simulink model "Noa_Nofusion_angle"  (R2020b)
settings: Solver=FixedStepDiscrete  StartTime=0.0  StopTime=Inf  FixedStep=0.01  RelTol=1e-3
PostLoadFcn:
  | if any(exist('dsrtsu_mdlpostloadfcn', 'file') ~= 0), dsrtsu_mdlpostloadfcn('Execute', bdroot); end
InitFcn:
  | , if any(exist('rtifpga_mdlclblib', 'file') ~= 0), rtifpga_mdlclblib('Init', bdroot); end,
  | , if any(exist('dsmpb_private', 'file') ~= 0), dsmpb_private('dsmpb_mdlclblib', 'Init', bdroot); end,
undefined symbols (not defined in the file): ACC_TimeGap_DecSetSwt, ACC_TimeGap_IncSetSwt, AccelPedalPosn, AccelPedalPosnVldty, AccelPedlPosnDiagc, AccPedalOverride, ACU_ShiftInProgress, ADAS_Posn_CurLane, AESSwtReq, ALC_SwtReq, BrkPedalSts, CC_ACC_CANCEL_OFFSwt, CC_ACC_CRUISE_OFFSwt, CC_ACC_DecSetSpd_SetSwt, CC_ACC_IncSetSpd_ResuSwt, CC_ACCSwtErr, CharSpd_ms, CSA_NODE, CURRENT_GEAR, CurrentGearValid, DiscIntNeverNeededParam, DrvDoorSts, DrvSBR, DrvTrqReqOvld, ECMACCInterface, ECMRespACC, ELKSwtReq, EngLimpHomeSts, EngSpd, EngState, EngState_PHEV, EngTrqMaxActSpd, EngTrqMinAct, EPS_DrvInpTrqVal_HighReslolution, EPS_FailSts, EPS_LKATorqOvrlDlvd, EPS_LKATorqOvrlDlvdVld, EPS_LKATrqOvlDlvdSts, EPS_SteerMod, EPS_TrqSnsrSts, EQ4_APPINFO, EQ4_LA_ELEM, EQ4_LA_HDR, EQ4_LAP_ELEM, EQ4_LAP_HDR, EQ4_LH_ELEM, EQ4_LH_HDR, EQ4_LRE_ELEM, EQ4_LRE_HDR, ESS_PedSwtReq, ESS_VehSwtReq, FFogLmpSts_F_Pbox, FLWheelDriveDirection, FLWheelSpd, FrntWiprSwtSts, FrntWshrSwtSts, FRWheelDriveDirection, FRWheelSpd, HazardLmpSwtSts, HCU_AccelPedalPosn_Diag ... (+151)
libraries: simulink x138, dsmpblib x33, canfdmsglib x10
(part 4 of 17)

== system Noa_Nofusion_angle/Common ==
  note: VIE
      | (VehicleInfomationEvaluation)
  note: CAL
      | (ConfigurationCalibration)
  note: DMS
      | (DriverMonitorSystem)
  note: EHR
      | (ElectronicHorizonReconstructor)
  IfCANBus : Inport
  function : TriggerPort  TriggerType=function-call  VariantControl=Variant
  Bus Assignment1 : BusAssignment  AssignedSignals=SteerWheelAngSign,SteerWheelAng,SteerWheelSpd,SAS_Sts
  Bus Assignment2 : BusAssignment  AssignedSignals=FLWheelSpd,FRWheelSpd,RLWheelSpd,RRWheelSpd,FLWheelDriveDirection,FRWheelDriveDirection,RLWheelDriveDirection,RRWheelDriveDirection,VehStandstill
  Bus Assignment3 : BusAssignment  AssignedSignals=VehLgtAccel,VehYawRate
  Bus Creator : BusCreator  Inputs=11
  Bus Creator2 : BusCreator  Commented=on  Inputs=6
  Bus Creator3 : BusCreator  Inputs=4
  Bus Creator4 : BusCreator  Inputs=3
  Bus Selector : BusSelector  OutputSignals=DMS_NODE.DMS_FD1_MSG.DMSSts,DMS_NODE.DMS_FD1_MSG.HeadDetn,DMS_NODE.DMS_FD1_MSG.DistrctnLvl_ACC,DMS_NODE.DMS_FD1_MSG.DistrctnLvlQlty_ACC,DMS_NODE.DMS_FD1_MSG.DrowsnsLvl_ACC
  Bus Selector2 : BusSelector  OutputSignals=ESP_NODE.ESP_FD3_MSG.FLWheelSpd,ESP_NODE.ESP_FD3_MSG.FRWheelSpd,ESP_NODE.ESP_FD3_MSG.RLWheelSpd,ESP_NODE.ESP_FD3_MSG.RRWheelSpd,ESP_NODE.ESP_FD3_MSG.FLWheelDriveDirection,ESP_NODE.ESP_FD3_MSG.FRWheelDriveDirection,ESP_NODE.ESP_FD3_MSG.RLWheelDriveDirection,ESP_NODE.ESP_FD3_MSG.RRWheelDriveDirection,ESP_NODE.ESP_FD2_MSG.VehStandstill
  Bus Selector3 : BusSelector  OutputSignals=CSA_NODE.CSA2_MSG.SteerWheelAngSign,CSA_NODE.CSA2_MSG.SteerWheelAng,CSA_NODE.CSA2_MSG.SteerWheelSpd,CSA_NODE.CSA2_MSG.SAS_Sts
  Bus Selector4 : BusSelector  OutputSignals=ABM_NODE.ABM2_MSG.VehLgtAccel,ABM_NODE.ABM2_MSG.VehYawRate
  Bus Selector8 : BusSelector  Commented=on  OutputSignals=ESP_NODE.ESP_FD2_MSG.VehSpd
  CAL : Subsystem
  Constant1 : Constant  Value=0  OutDataTypeStr=Bus: VCAN_CSA_MSG_BUS
  Constant2 : Constant  Value=0  OutDataTypeStr=Bus: VCAN_ABM_MSG_BUS
  Constant3 : Constant  Value=0  OutDataTypeStr=Bus: VCAN_ESP_MSG_BUS
  DMS : ModelReference  Commented=on  ModelNameDialog=PubIfCommonDMS_MDL.slx  SimulationMode=Normal  ModelReferenceVersion=3.0
  Data Outport : dsmpblib/Data Outport  Priority=-10000
      settings: SourceProductName=dSPACE Model Interface Blockset
  Data Outport1 : dsmpblib/Data Outport  Priority=-10000
      settings: SourceProductName=dSPACE Model Interface Blockset
  EHR : ModelReference  Commented=on  ModelNameDialog=PubIfCommonEHRV2_MDL_New.slx  SimulationMode=Normal  ModelReferenceVersion=1.4
  Ground : Ground  Commented=on
  S-Function Builder : S-Function  Commented=on  FunctionName=SWC_VIE  SFunctionModules=SWC_VIE_wrapper PubIfCommonVIE_MDL  SFunctionDeploymentMode=off  EnableBusSupport=off  mask(S-Function Builder){}
      mask help: Simulink:masks:SFunctionBuilder_MD
      mask init:
      | val = [[.9  0.75 0.75 1 1 .9 .9 1]',[1 1 0.75 0.75 .9 .9 1 .9]'];try , sys = get_param(gcb,'SfunBuilderFcnName');if isempty(sys), sys = get_param(gcb,'FunctionName'); end,catch, sys = get_param(gcb,'FunctionName'); end
      settings: CopyFcn=set_param(gcbh,'LinkStatus','none')  OpenFcn=sfunctionwizard(gcbh)
      mask Display: plot(val(:,1),val(:,2)),disp(sys),port_label('input',1,'arg_VIE_VCAN_ESP'),port_label('input',2,'arg_VIE_VCAN_CSA'),port_label('input',3,'arg_VIE_VCAN_ABM'),port_label('output',1,'arg_axvRefMs2'),port_label('output',2,'arg_vxvRefMs'),port_label('output',3,'arg_axvRoadSlopeMs2'),port_label('output',4,'arg_axRefMs2'),port_label('output',5,'arg_axRefDt'),port_label('output',6,'arg_psiDtOpt'),port_label('output',7,'arg_ayvRefMs2'),port_label('output',8,'arg_alpSideSlipAngle'),port_label('output',9,'arg_kapTraj'),port_label('output',10,'arg_alpSumSlideCurveness'),port_label('output',11,'arg_SteerAngleOffset_deg')
  Subsystem1 : Subsystem  Commented=on
  Subsystem2 : Subsystem  Commented=on
  Subsystem3 : Subsystem  Commented=on
  Subsystem4 : Subsystem  Commented=on
  Subsystem5 : Subsystem  Commented=on
  Subsystem6 : Subsystem  Commented=on
  Subsystem7 : Subsystem
  VIE : ModelReference  ModelNameDialog=PubIfCommonVIE_MDL.slx  SimulationMode=Normal  ModelReferenceVersion=3.6
  IfCALBus : Outport
  IfDMSBus : Outport  Port=2
  IfVIEBus : Outport  Port=3
  IfEHRBus : Outport  Port=4
  wires:
  VIE/8 -> Bus Creator/8  "alpSideSlipAngle"
  Bus Creator3/1 -> IfCALBus/1  "IfCALBus"
  VIE/6 -> Bus Creator/6  "psiDtOpt"
  CAL/2(CAL_AEB_CONFIG) -> Bus Creator3/2  "CAL_AEB_CONFIG"
  VIE/1 -> Bus Creator/1  "axvRefMs2"
  VIE/2 -> Bus Creator/2  "vxvRefMs"
  VIE/9 -> Bus Creator/9  "kapTraj"
  Bus Creator/1 -> IfVIEBus/1, Data Outport/1  "IfVIEBus"
  Bus Creator2/1 -> IfEHRBus/1  "IfEHRBus"
  Subsystem7/2(DMS_DrowsnsSts) -> Bus Creator4/2  "DrowsnsSts"
  Subsystem7/1(DMS_DistractnSts) -> Bus Creator4/1  "DistractnSts"
  IfCANBus/1 -> [IfCANBus]
  [IfCANBus] -> Bus Selector/1
  VIE/4 -> Bus Creator/4  "axRefMs2"
  Bus Creator4/1 -> IfDMSBus/1, Data Outport1/1  "IfDMSBus"
  VIE/7 -> Bus Creator/7  "ayvRefMs2"
  CAL/3(NvMReadWriteU8) -> Bus Creator3/3  "NvMReadWriteU8"
  CAL/4(CAL_AHBC_CONFIG) -> Bus Creator3/4  "CAL_AHBC_CONFIG"
  Subsystem7/3(DMS_DriverSts) -> Bus Creator4/3  "DriverSts"
  VIE/10 -> Bus Creator/10  "alpSumSlideCurveness"
  VIE/3 -> Bus Creator/3  "axvRoadSlopeMs2"
  VIE/5 -> Bus Creator/5  "axRefDt"
  CAL/1(CAL_VSM_CONFIG) -> Bus Creator3/1  "CAL_VSM_CONFIG"
  VIE/11 -> Bus Creator/11  "SteerAngleOffset_deg"
  Subsystem1/1(EHRV2_VCAN_POSN) -> EHR/1
  Subsystem3/1(EHRV2_VCAN_STUB) -> EHR/3
  Subsystem5/1(EHRV2_VCAN_SEG) -> EHR/2
  Subsystem4/1(EHRV2_VCAN_PROFLONG) -> EHR/5
  Subsystem2/1(EHRV2_VCAN_PROFSHORT) -> EHR/4
  Subsystem6/1(EHRV2_VCAN_META) -> EHR/6
  Bus Selector8/1 -> EHR/7  "<VehSpd>"
  Ground/1 -> EHR/8
  [IfCANBus] -> Bus Selector8/1, Subsystem6/1(In1), Subsystem4/1(In1), Subsystem2/1(In1), Subsystem3/1(In1), Subsystem5/1(In1), Subsystem1/1(In1)
  Bus Selector/1 -> Subsystem7/1(DMSSts)  "<DMSSts>"
  Bus Selector/2 -> Subsystem7/2(HeadDetn)  "<HeadDetn>"
  Bus Selector/3 -> Subsystem7/3(DistrctnLvl_ACC)  "<DistrctnLvl_ACC>"
  Bus Selector/4 -> Subsystem7/4(DistrctnLvlQlty_ACC)  "<DistrctnLvlQlty_ACC>"
  Bus Selector/5 -> Subsystem7/5(DrowsnsLvl_ACC)  "<DrowsnsLvl_ACC>"
  [IfCANBus] -> Bus Selector4/1, Bus Selector3/1, Bus Selector2/1
  EHR/1 -> Bus Creator2/1  "EHRV2_HDR"
  EHR/2 -> Bus Creator2/2  "EHRV2_HutHandshake"
  EHR/3 -> Bus Creator2/3  "EHRV2_ROAD_ROI"
  EHR/4 -> Bus Creator2/4  "EHRV2_ROAD_INFO"
  EHR/5 -> Bus Creator2/5  "EHRV2_NAV_INFO"
  EHR/6 -> Bus Creator2/6  "EHRV2_DYNAMIC_INFO"
  Constant3/1 -> Bus Assignment2/1
  Bus Selector2/1 -> Bus Assignment2/2  "<FLWheelSpd>"
  Bus Selector2/2 -> Bus Assignment2/3  "<FRWheelSpd>"
  Bus Selector2/3 -> Bus Assignment2/4  "<RLWheelSpd>"
  Bus Selector2/4 -> Bus Assignment2/5  "<RRWheelSpd>"
  Bus Selector2/5 -> Bus Assignment2/6  "<FLWheelDriveDirection>"
  Bus Selector2/6 -> Bus Assignment2/7  "<FRWheelDriveDirection>"
  Bus Selector2/7 -> Bus Assignment2/8  "<RLWheelDriveDirection>"
  Bus Selector2/8 -> Bus Assignment2/9  "<RRWheelDriveDirection>"
  Bus Selector2/9 -> Bus Assignment2/10  "<VehStandstill>"
  Bus Assignment2/1 -> VIE/1
  Constant1/1 -> Bus Assignment1/1
  Bus Selector3/1 -> Bus Assignment1/2  "<SteerWheelAngSign>"
  Bus Selector3/2 -> Bus Assignment1/3  "<SteerWheelAng>"
  Bus Selector3/3 -> Bus Assignment1/4  "<SteerWheelSpd>"
  Bus Selector3/4 -> Bus Assignment1/5  "<SAS_Sts>"
  Bus Assignment1/1 -> VIE/2
  Constant2/1 -> Bus Assignment3/1
  Bus Selector4/1 -> Bus Assignment3/2  "<VehLgtAccel>"
  Bus Selector4/2 -> Bus Assignment3/3  "<VehYawRate>"
  Bus Assignment3/1 -> VIE/3

== system Noa_Nofusion_angle/Control1 ==
  note: VMC-LAT
      | (LateralControl)
  note: VMC-LON
      | (LongtitudeControl)
  IfVCANBus : Inport  OutDataTypeStr=Bus: VCAN_BUS
  IfVSMBus : Inport  Port=2
  IfTOSBus : Inport  Port=3
  IfRFMBus : Inport  Port=4
  IfEHRBus : Inport  Port=5
  IfVIEBus : Inport  Port=6
  IfRoadBus : Inport  Port=7
  IfPlanbus : Inport  Port=8
  roadwidth : Inport  Port=9
  function : TriggerPort  TriggerType=function-call  VariantControl=Variant
  Bus Assignment : BusAssignment  AssignedSignals=dCurrentLaneWidth
  Bus Assignment1 : BusAssignment  AssignedSignals=CURRENT_GEAR,SHIFT_IN_PROGRESS
  Bus Assignment2 : BusAssignment  AssignedSignals=NoBrkForce,VehStandstill
  Bus Assignment4 : BusAssignment  AssignedSignals=ACU_ShiftInProgress,HCU_PTDrvMod,TotWheelTrq,MinPsblWheelTrq
  Bus Creator1 : BusCreator  Inputs=3
  Bus Creator2 : BusCreator  Inputs=4
  Bus Creator3 : BusCreator  Inputs=4
  Bus Selector : BusSelector  OutputSignals=PLAN_ACCPLAN,PLAN_Longctrl_DecelToStopReq
  Bus Selector1 : BusSelector  OutputSignals=vxvRefMs,axvRefMs2,ayvRefMs2,kapTraj,alpSideSlipAngle,psiDtOpt,SteerAngleOffset_deg
  Bus Selector11 : BusSelector  OutputSignals=RFM_ROAD
  Bus Selector13 : BusSelector  OutputSignals=DCT_NODE.DCT5_MSG.CURRENT_GEAR,DCT_NODE.DCT5_MSG.SHIFT_IN_PROGRESS
  Bus Selector2 : BusSelector  OutputSignals=EPS_NODE.EPS_FD1_MSG.EPS_SteerMod,EPS_NODE.EPS_FD1_MSG.EPS_DrvInpTrqVal_HighReslolution,EPS_NODE.EPS_FD1_MSG.EPS_LKATorqOvrlDlvd,EPS_NODE.EPS_FD1_MSG.EPS_LKATorqOvrlDlvdVld
  Bus Selector3 : BusSelector  OutputSignals=vxvRefMs,axvRoadSlopeMs2,axRefMs2,alpSideSlipAngle,axRefDt
  Bus Selector4 : BusSelector  OutputSignals=CSA_NODE.CSA2_MSG.SteerWheelAng,CSA_NODE.CSA2_MSG.SteerWheelAngSign,CSA_NODE.CSA2_MSG.SteerWheelSpd,CSA_NODE.CSA2_MSG.SteerWheelSpdSign
  Bus Selector5 : BusSelector  OutputSignals=ESP_NODE.ESP_FD2_MSG.NoBrkForce,ESP_NODE.ESP_FD2_MSG.VehStandstill
  Bus Selector6 : BusSelector  OutputSignals=VSM_LAT_CTRL
  Bus Selector7 : BusSelector  OutputSignals=HCU_NODE.HCU_FD1_MSG.ACU_ShiftInProgress,HCU_NODE.HCU_FD3_MSG.HCU_PTDrvMod,HCU_NODE.HCU_FD1_MSG.TotWheelTrq,HCU_NODE.HCU_FD1_MSG.MinPsblWheelTrq
  Bus Selector8 : BusSelector  OutputSignals=VSM_LON_CTRL
  Bus Creator : BusCreator  Inputs=4
  Constant1 : Constant  Value=0  OutDataTypeStr=Bus: VCAN_DCT_MSG_BUS
  Constant3 : Constant  Value=0  OutDataTypeStr=Bus: VCAN_ESP_MSG_BUS
  Constant4 : Constant  Value=0  OutDataTypeStr=Bus: VCAN_HCU_MSG_BUS
  Data Type Conversion : DataTypeConversion
  LATC : ModelReference  ModelNameDialog=PubIfControlLATC_MDL.slx  SimulationMode=Normal  ModelReferenceVersion=3.279
  LON : ModelReference  ModelNameDialog=PubIfControlLONC_MDL.slx  SimulationMode=Normal  ModelReferenceVersion=3.54
  Signal Copy : SignalConversion  OverrideOpt=off
  Subsystem : Subsystem
  Terminator : Terminator
  Terminator2 : Terminator
  IfLONBus : Outport
  IfLATBus : Outport  Port=2
  wires:
  IfVIEBus/1 -> Bus Selector3/1, Bus Selector1/1
  Bus Creator1/1 -> IfLONBus/1  "IfLONBus"
  IfVCANBus/1 -> Bus Selector7/1, Subsystem/1(In1), Bus Selector13/1, Bus Selector5/1, Bus Selector4/1, Bus Selector2/1
  IfVSMBus/1 -> Bus Selector8/1, Bus Selector6/1
  IfRoadBus/1 -> Bus Selector11/1
  Bus Selector11/1 -> Bus Assignment/1  "<RFM_ROAD>"
  Bus Selector1/7 -> LATC/8  "<SteerAngleOffset_deg>"
  Bus Selector2/3 -> Bus Creator2/3  "<EPS_LKATorqOvrlDlvd>"
  Bus Selector2/2 -> Bus Creator2/2  "<EPS_DrvInpTrqVal_HighReslolution>"
  Bus Selector2/4 -> Bus Creator2/4  "<EPS_LKATorqOvrlDlvdVld>"
  Bus Selector2/1 -> Bus Creator2/1  "<EPS_SteerMod>"
  Bus Creator2/1 -> LATC/9
  Bus Selector4/2 -> Bus Creator3/2  "<SteerWheelAngSign>"
  Bus Selector4/3 -> Bus Creator3/3  "<SteerWheelSpd>"
  Bus Selector4/1 -> Bus Creator3/1  "<SteerWheelAng>"
  Bus Selector4/4 -> Bus Creator3/4  "<SteerWheelSpdSign>"
  Bus Creator3/1 -> LATC/10
  LON/1 -> Bus Creator1/1  "LONC_CTRL_OUT"
  LON/3 -> Bus Creator1/3  "LONC_VLC_InternalAcc"
  Bus Selector6/1 -> LATC/1  "<VSM_LAT_CTRL>"
  Bus Selector1/1 -> LATC/2  "<vxvRefMs>"
  Bus Selector1/2 -> LATC/3  "<axvRefMs2>"
  Bus Selector1/3 -> LATC/4  "<ayvRefMs2>"
  Bus Selector1/4 -> LATC/5  "<kapTraj>"
  Bus Selector1/5 -> Signal Copy/1  "<alpSideSlipAngle>"
  Bus Selector1/6 -> LATC/7  "<psiDtOpt>"
  IfPlanbus/1 -> Bus Selector/1
  Bus Selector3/1 -> LON/1  "<vxvRefMs>"
  Bus Selector3/2 -> LON/2  "<axvRoadSlopeMs2>"
  Bus Selector3/3 -> LON/3  "<axRefMs2>"
  Bus Selector3/4 -> LON/4  "<alpSideSlipAngle>"
  Bus Selector3/5 -> LON/5  "<axRefDt>"
  Bus Selector8/1 -> LON/10  "<VSM_LON_CTRL>"
  Bus Selector/1 -> LON/11  "<PLAN_ACCPLAN>"
  IfRFMBus/1 -> Terminator/1
  IfTOSBus/1 -> Terminator2/1
  Bus Selector/2 -> LON/12  "<PLAN_Longctrl_DecelToStopReq>"
  Constant3/1 -> Bus Assignment2/1
  Bus Assignment2/1 -> LON/6
  Bus Selector5/1 -> Bus Assignment2/2  "<NoBrkForce>"
  Bus Selector5/2 -> Bus Assignment2/3  "<VehStandstill>"
  Constant1/1 -> Bus Assignment1/1
  Bus Selector13/1 -> Bus Assignment1/2  "<CURRENT_GEAR>"
  Bus Selector13/2 -> Bus Assignment1/3  "<SHIFT_IN_PROGRESS>"
  Bus Assignment1/1 -> LON/7
  LON/2 -> Bus Creator1/2  "LONC_Hybrid_CTRL_OUT"
  Constant4/1 -> Bus Assignment4/1
  Subsystem/1(Out1) -> LON/8
  Bus Assignment4/1 -> LON/9
  Bus Selector7/1 -> Bus Assignment4/2  "<ACU_ShiftInProgress>"
  Bus Selector7/3 -> Bus Assignment4/4  "<TotWheelTrq>"
  Bus Selector7/2 -> Bus Assignment4/3  "<HCU_PTDrvMod>"
  Bus Selector7/4 -> Bus Assignment4/5  "<MinPsblWheelTrq>"
  Data Type Conversion/1 -> Bus Assignment/2
  Bus Assignment/1 -> LATC/11
  roadwidth/1 -> [roadwidth], Data Type Conversion/1
  LATC/1 -> Bus Creator/1  "IfLATBus"
  LATC/2 -> Bus Creator/2
  LATC/3 -> Bus Creator/3
  LATC/4 -> Bus Creator/4
  Bus Creator/1 -> IfLATBus/1
  Signal Copy/1 -> LATC/6

== system Noa_Nofusion_angle/EQ4_Lane_Pack1 ==
  In1 : Inport
  Bus Assignment : BusAssignment  AssignedSignals=LA_Zero_byte,LA_Protocol_Version,LA_Sync_ID,LA_Adjacent_Count
  Bus Assignment1 : BusAssignment  AssignedSignals=EQ4_LH_HDR,EQ4_LH_ELEM,EQ4_APPINFO.APP_SyncTs
  Bus Assignment2 : BusAssignment  AssignedSignals=EQ4_LRE_HDR,EQ4_LRE_ELEM
  Bus Assignment3 : BusAssignment  AssignedSignals=EQ4_LA_HDR,EQ4_LA_ELEM
  Bus Assignment4 : BusAssignment  AssignedSignals=LRE_Zero_byte,Reserved_1,LRE_CRC,LRE_Protocol_Version,LRE_Sync_ID,LRE_Count,LRE_Header_Buffer
  Bus Assignment5 : BusAssignment  AssignedSignals=LAP_Zero_byte,LAP_Protocol_Version,LAP_Sync_ID,LAP_Is_Construction_Area,LAP_Buffer_C0,LAP_INTP_Available,LAP_INTP_Count,LAP_Exit_Merge_Available,LAP_Is_Highway_Merge_Left,LAP_Is_Highway_Merge_Right,LAP_Is_Highway_Exit_Left,LAP_Is_Highway_Exit_Right,LAP_Vertical_Surface_Available,LAP_Vertical_Surface_VR_End,Reserved_1,LAP_Vertical_Surface_C0,LAP_Vertical_Surface_C1,LAP_Vertical_Surface_C2,LAP_Vertical_Surface_C3,LAP_Path_Pred_CRC,LAP_Path_Pred_Available,LAP_Path_Pred_First_Valid,LAP_Path_Pred_Second_Valid,LAP_Path_Pred_Half_Width,LAP_Path_Pred_Conf,LAP_Is_Triggered_SDM_Model,Reserved_2,LAP_Path_Pred_First_VR_End,LAP_Path_Pred_second_VR_End,Reserved_3,LAP_Path_Pred_First_C0,LAP_Path_Pred_First_C1,LAP_Path_Pred_First_C2,LAP_Path_Pred_First_C3,LAP_Path_Pred_Second_C0,LAP_Path_Pred_Second_C1,LAP_Path_Pred_Second_C2,LAP_Path_Pred_Second_C3
  Bus Assignment6 : BusAssignment  AssignedSignals=LH_Zero_byte,LH_Protocol_Version,LH_Sync_ID,LH_Lanes_Count,Reserved_1,LH_Estimated_Width,Reserved_2
  Bus Assignment7 : BusAssignment  AssignedSignals=EQ4_LAP_HDR,EQ4_LAP_ELEM
  Bus Selector : BusSelector  OutputSignals=EQ4_LA.EQ4_LA_HDR,EQ4_LA.EQ4_LA_ELEM,EQ4_LA.EQ4_APPINFO.H
  Bus Selector1 : BusSelector  OutputSignals=EQ4_LH.EQ4_LH_HDR,EQ4_LH.EQ4_LH_ELEM,EQ4_LH.EQ4_APPINFO.H
  Bus Selector2 : BusSelector  OutputSignals=EQ4_LRE.EQ4_LRE_HDR,EQ4_LRE.EQ4_LRE_ELEM,EQ4_LRE.EQ4_APPINFO.H
  Bus Selector3 : BusSelector  OutputSignals=LA_Zero_byte,LA_Protocol_Version,LA_Sync_ID,LA_Adjacent_Count
  Bus Selector4 : BusSelector  OutputSignals=LRE_Zero_byte,Reserved_1,LRE_CRC,LRE_Protocol_Version,LRE_Sync_ID,LRE_Count,LRE_Header_Buffer
  Bus Selector5 : BusSelector  OutputSignals=LH_Zero_byte,LH_Protocol_Version,LH_Sync_ID,LH_Lanes_Count,Reserved_1,LH_Estimated_Width,Reserved_2
  Bus Selector6 : BusSelector  OutputSignals=EQ4_LAP.EQ4_LAP_HDR,EQ4_LAP.EQ4_LAP_ELEM,EQ4_LAP.EQ4_APPINFO.H
  Bus Selector7 : BusSelector  OutputSignals=LAP_Zero_byte,LAP_Protocol_Version,LAP_Sync_ID,LAP_Is_Construction_Area,LAP_Buffer_C0,LAP_INTP_Available,LAP_INTP_Count,LAP_Exit_Merge_Available,LAP_Is_Highway_Merge_Left,LAP_Is_Highway_Merge_Right,LAP_Is_Highway_Exit_Left,LAP_Is_Highway_Exit_Right,LAP_Vertical_Surface_Available,LAP_Vertical_Surface_VR_End,Reserved_1,LAP_Vertical_Surface_C0,LAP_Vertical_Surface_C1,LAP_Vertical_Surface_C2,LAP_Vertical_Surface_C3,LAP_Path_Pred_CRC,LAP_Path_Pred_Available,LAP_Path_Pred_First_Valid,LAP_Path_Pred_Second_Valid,LAP_Path_Pred_Half_Width,LAP_Path_Pred_Conf,LAP_Is_Triggered_SDM_Model,Reserved_2,LAP_Path_Pred_First_VR_End,LAP_Path_Pred_second_VR_End,Reserved_3,LAP_Path_Pred_First_C0,LAP_Path_Pred_First_C1,LAP_Path_Pred_First_C2,LAP_Path_Pred_First_C3,LAP_Path_Pred_Second_C0,LAP_Path_Pred_Second_C1,LAP_Path_Pred_Second_C2,LAP_Path_Pred_Second_C3
  Constant1 : Constant  Value=0  OutDataTypeStr=Bus: EQ4_LA_BUS
  Constant2 : Constant  Value=0  OutDataTypeStr=Bus: EQ4_LH_BUS
  Constant3 : Constant  Value=0  OutDataTypeStr=Bus: EQ4_LRE_BUS
  Constant4 : Constant  Value=0  OutDataTypeStr=Bus: EQ4_LA_HDR_BUS
  Constant5 : Constant  Value=0  OutDataTypeStr=Bus: EQ4_LRE_HDR_BUS
  Constant6 : Constant  Value=0  OutDataTypeStr=Bus: EQ4_LAP_BUS
  Constant7 : Constant  Value=0  OutDataTypeStr=Bus: EQ4_LH_HDR_BUS
  Constant8 : Constant  Value=0  OutDataTypeStr=Bus: EQ4_LAP_HDR_BUS
  Data Type Conversion{,1..4} (5 alike) : DataTypeConversion
  For Each Subsystem1 : Subsystem  TreatAsAtomicUnit=on
  For Each Subsystem2 : Subsystem  TreatAsAtomicUnit=on
  For Each Subsystem3 : Subsystem  TreatAsAtomicUnit=on
  For Each Subsystem4 : Subsystem  TreatAsAtomicUnit=on
  EQ4_LAP : Outport
  EQ4_LA : Outport  Port=2
  EQ4_LH : Outport  Port=3
  EQ4_LRE : Outport  Port=4
  wires:
  In1/1 -> Bus Selector2/1, Bus Selector1/1, Bus Selector6/1, Bus Selector/1
  Bus Assignment2/1 -> EQ4_LRE/1  "mcuEQ4_LRE"
  Constant2/1 -> Bus Assignment1/1
  Bus Assignment1/1 -> EQ4_LH/1  "mcuEQ4_LH"
  Constant3/1 -> Bus Assignment2/1
  Bus Assignment3/1 -> EQ4_LA/1  "mcuEQ4_LA"
  Bus Selector/1 -> Bus Selector3/1  "<EQ4_LA_HDR>"
  Bus Selector/2 -> For Each Subsystem3/1(In1)  "<EQ4_LA_ELEM>"
  Bus Selector1/1 -> Bus Selector5/1  "<EQ4_LH_HDR>"
  Bus Selector1/2 -> For Each Subsystem1/1(In1)  "<EQ4_LH_ELEM>"
  Bus Selector2/1 -> Bus Selector4/1  "<EQ4_LRE_HDR>"
  Bus Selector2/2 -> For Each Subsystem2/1(In1)  "<EQ4_LRE_ELEM>"
  Constant1/1 -> Bus Assignment3/1
  Constant4/1 -> Bus Assignment/1
  Bus Assignment/1 -> Bus Assignment3/2
  Bus Selector3/1 -> Bus Assignment/2  "<LA_Zero_byte>"
  Bus Selector3/2 -> Bus Assignment/3  "<LA_Protocol_Version>"
  Bus Selector3/4 -> Bus Assignment/5  "<LA_Adjacent_Count>"
  Constant5/1 -> Bus Assignment4/1
  Bus Selector4/6 -> Bus Assignment4/7  "<LRE_Count>"
  Bus Selector4/7 -> Bus Assignment4/8  "<LRE_Header_Buffer>"
  Bus Selector4/4 -> Bus Assignment4/5  "<LRE_Protocol_Version>"
  Bus Selector4/3 -> Bus Assignment4/4  "<LRE_CRC>"
  Bus Selector4/2 -> Bus Assignment4/3  "<Reserved_1>"
  Bus Selector4/1 -> Bus Assignment4/2  "<LRE_Zero_byte>"
  Bus Assignment4/1 -> Bus Assignment2/2
  Constant7/1 -> Bus Assignment6/1
  Bus Assignment6/1 -> Bus Assignment1/2
  Bus Selector5/6 -> Bus Assignment6/7  "<LH_Estimated_Width>"
  Bus Selector5/5 -> Bus Assignment6/6  "<Reserved_1>"
  Bus Selector5/7 -> Bus Assignment6/8  "<Reserved_2>"
  Bus Selector5/4 -> Bus Assignment6/5  "<LH_Lanes_Count>"
  Bus Selector5/2 -> Bus Assignment6/3  "<LH_Protocol_Version>"
  Bus Selector5/1 -> Bus Assignment6/2  "<LH_Zero_byte>"
  For Each Subsystem1/1(Out1) -> Bus Assignment1/3
  For Each Subsystem2/1(Out1) -> Bus Assignment2/3
  For Each Subsystem3/1(Out1) -> Bus Assignment3/3
  Bus Selector1/3 -> Data Type Conversion2/1, Data Type Conversion/1  "<H>"
  Data Type Conversion/1 -> Bus Assignment1/4
  Bus Selector/3 -> Data Type Conversion1/1  "<H>"
  Data Type Conversion1/1 -> Bus Assignment/4
  Data Type Conversion2/1 -> Bus Assignment6/4
  Data Type Conversion3/1 -> Bus Assignment4/6
  Bus Selector2/3 -> Data Type Conversion3/1  "<H>"
  Data Type Conversion4/1 -> Bus Assignment5/4
  For Each Subsystem4/1(Out1) -> Bus Assignment7/3
  Bus Assignment5/1 -> Bus Assignment7/2
  Constant8/1 -> Bus Assignment5/1
  Constant6/1 -> Bus Assignment7/1
  Bus Selector6/2 -> For Each Subsystem4/1(In1)  "<EQ4_LAP_ELEM>"
  Bus Assignment7/1 -> EQ4_LAP/1  "mcuEQ4_LAP"
  Bus Selector6/3 -> Data Type Conversion4/1  "<H>"
  Bus Selector6/1 -> Bus Selector7/1  "<EQ4_LAP_HDR>"
  Bus Selector7/1 -> Bus Assignment5/2  "<LAP_Zero_byte>"
  Bus Selector7/2 -> Bus Assignment5/3  "<LAP_Protocol_Version>"
  Bus Selector7/4 -> Bus Assignment5/5  "<LAP_Is_Construction_Area>"
  Bus Selector7/5 -> Bus Assignment5/6  "<LAP_Buffer_C0>"
  Bus Selector7/6 -> Bus Assignment5/7  "<LAP_INTP_Available>"
  Bus Selector7/7 -> Bus Assignment5/8  "<LAP_INTP_Count>"
  Bus Selector7/8 -> Bus Assignment5/9  "<LAP_Exit_Merge_Available>"
  Bus Selector7/9 -> Bus Assignment5/10  "<LAP_Is_Highway_Merge_Left>"
  Bus Selector7/10 -> Bus Assignment5/11  "<LAP_Is_Highway_Merge_Right>"
  Bus Selector7/11 -> Bus Assignment5/12  "<LAP_Is_Highway_Exit_Left>"
  Bus Selector7/12 -> Bus Assignment5/13  "<LAP_Is_Highway_Exit_Right>"
  Bus Selector7/13 -> Bus Assignment5/14  "<LAP_Vertical_Surface_Available>"
  Bus Selector7/14 -> Bus Assignment5/15  "<LAP_Vertical_Surface_VR_End>"
  Bus Selector7/15 -> Bus Assignment5/16  "<Reserved_1>"
  Bus Selector7/16 -> Bus Assignment5/17  "<LAP_Vertical_Surface_C0>"
  Bus Selector7/17 -> Bus Assignment5/18  "<LAP_Vertical_Surface_C1>"
  Bus Selector7/18 -> Bus Assignment5/19  "<LAP_Vertical_Surface_C2>"
  Bus Selector7/19 -> Bus Assignment5/20  "<LAP_Vertical_Surface_C3>"
  Bus Selector7/20 -> Bus Assignment5/21  "<LAP_Path_Pred_CRC>"
  Bus Selector7/21 -> Bus Assignment5/22  "<LAP_Path_Pred_Available>"
  Bus Selector7/22 -> Bus Assignment5/23  "<LAP_Path_Pred_First_Valid>"
  Bus Selector7/23 -> Bus Assignment5/24  "<LAP_Path_Pred_Second_Valid>"
  Bus Selector7/24 -> Bus Assignment5/25  "<LAP_Path_Pred_Half_Width>"
  Bus Selector7/25 -> Bus Assignment5/26  "<LAP_Path_Pred_Conf>"
  Bus Selector7/26 -> Bus Assignment5/27  "<LAP_Is_Triggered_SDM_Model>"
  Bus Selector7/27 -> Bus Assignment5/28  "<Reserved_2>"
  Bus Selector7/28 -> Bus Assignment5/29  "<LAP_Path_Pred_First_VR_End>"
  Bus Selector7/29 -> Bus Assignment5/30  "<LAP_Path_Pred_second_VR_End>"
  Bus Selector7/30 -> Bus Assignment5/31  "<Reserved_3>"
  Bus Selector7/31 -> Bus Assignment5/32  "<LAP_Path_Pred_First_C0>"
  Bus Selector7/32 -> Bus Assignment5/33  "<LAP_Path_Pred_First_C1>"
  Bus Selector7/33 -> Bus Assignment5/34  "<LAP_Path_Pred_First_C2>"
  Bus Selector7/34 -> Bus Assignment5/35  "<LAP_Path_Pred_First_C3>"
  Bus Selector7/35 -> Bus Assignment5/36  "<LAP_Path_Pred_Second_C0>"
  Bus Selector7/36 -> Bus Assignment5/37  "<LAP_Path_Pred_Second_C1>"
  Bus Selector7/37 -> Bus Assignment5/38  "<LAP_Path_Pred_Second_C2>"
  Bus Selector7/38 -> Bus Assignment5/39  "<LAP_Path_Pred_Second_C3>"

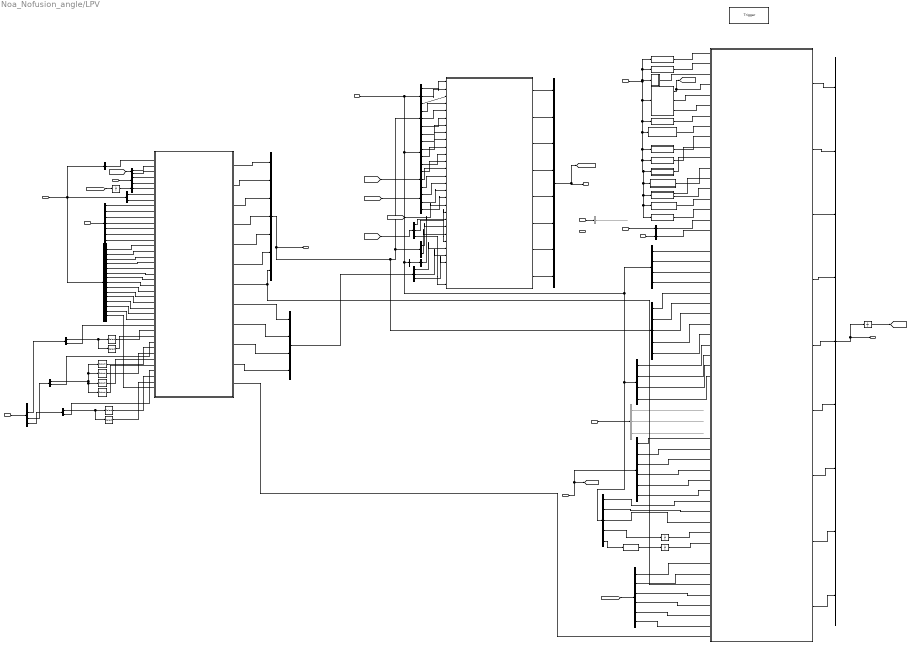
== system Noa_Nofusion_angle/LPV ==
  FaultRnk : Inport
  FaultTriggers : Inport  Port=2
  IfALLBus : Inport  Port=3
  IfCANBus : Inport  Port=4
  IfCALBus : Inport  Port=5
  IfDMSBus : Inport  Port=6
  IfEHRBus : Inport  Port=7
  IfVIEBus : Inport  Port=8
  IfEQ4Bus : Inport  Port=9
  RFM_LANES : Inport  Port=10
  function : TriggerPort  TriggerType=function-call  VariantControl=Variant
  ABM_Pack : Subsystem
  BCM_Pack : Subsystem
  Bus Creator : BusCreator  Inputs=9
  Bus Creator1 : BusCreator  Inputs=8
  Bus Creator3 : BusCreator  Inputs=4
  Bus Creator9 : BusCreator  Inputs=7
  Bus Selector : BusSelector  OutputSignals=LSM_UpdateCnt,LSM_TJA_ICA,LSM_HWA,LSM_LCK,LSM_ESS
  Bus Selector1 : BusSelector  OutputSignals=signal1.TOS_P0_TARGET_LINE
  Bus Selector10 : BusSelector  OutputSignals=LSM_HWA,LSM_ESS,LSM_UpdateCnt
  Bus Selector12 : BusSelector  OutputSignals=VSM_LON_CTRL
  Bus Selector13 : BusSelector  OutputSignals=LSM_PilotSPLDist,LSM_PilotSPL,LSM_PilotRoadSts
  Bus Selector14 : BusSelector  OutputSignals=PLAN_ALC_DECS
  Bus Selector15 : BusSelector  OutputSignals=EQ4_LA_ELEM,EQ4_LA_HDR
  Bus Selector16 : BusSelector  OutputSignals=PLAN_ACCPLAN,PLAN_DriverOffConditionFulfilled,PLAN_ALC_DECS,PLAN_DPC_ESS,PLAN_NOH_SetSpdAdjReq,PLAN_NOH_SetSpdAdjVal
  Bus Selector17 : BusSelector  OutputSignals=EQ4_LH_ELEM,EQ4_LH_HDR
  Bus Selector18 : BusSelector  OutputSignals=VSM_HMI,VSM_UOM_LC_BUS,MRCReq
  Bus Selector19 : BusSelector  OutputSignals=DriverSts
  Bus Selector2 : BusSelector  OutputSignals=vxvRefMs,kapTraj
  Bus Selector20 : BusSelector  OutputSignals=CAL_VSM_CONFIG
  Bus Selector21 : BusSelector  OutputSignals=lanebus.RFM_LINE_L1,lanebus.RFM_LINE_R1,lanebus.RFM_LINE_LB,lanebus.RFM_LINE_RB
  Bus Selector22 : BusSelector  Commented=on  OutputSignals=EHRV2_HDR,EHRV2_ROAD_ROI,EHRV2_ROAD_INFO
  Bus Selector23 : BusSelector  OutputSignals=axvRefMs2,vxvRefMs,axvRoadSlopeMs2,axRefDt,ayvRefMs2,kapTraj
  Bus Selector24 : BusSelector  OutputSignals=aebbus.AEB_IPHUT_INFO,aebbus.AEB_BRK_INFO,roadbus.RFM_TSR,latbus.LATC_IFCAngCmdReqValue,latbus.LATC_IFCFuncAngCmdReqFlag
  Bus Selector25 : BusSelector  OutputSignals=signal1.TOS_ACCP0,signal1.TOS_AEB_LONOBJ,signal1.TOS_ELK,signal1.TOS_LCKIE
  Bus Selector26 : BusSelector  OutputSignals=EQ4_LRE_ELEM,EQ4_LRE_HDR
  Bus Selector27 : BusSelector  OutputSignals=lanebus.RFM_LINE_L1,lanebus.RFM_LINE_R1,roadbus.RFM_TSR
  Bus Selector28 : BusSelector  OutputSignals=LONC_VLC_InternalAcc
  Bus Selector29 : BusSelector  OutputSignals=LSM_PilotSts,LSM_PilotTurnSwSts
  Bus Selector3 : BusSelector  OutputSignals=lanebus.RFM_LINE_L1,lanebus.RFM_LINE_R1,lanebus.RFM_LINE_L2,lanebus.RFM_LINE_R2,lanebus.RFM_LINE_L3,lanebus.RFM_LINE_R3,lanebus.RFM_LINE_CL,lanebus.RFM_LINE_LB,lanebus.RFM_LINE_RB,lanebus.RFM_LINE_PRED,lanebus.RFM_LINEF_LB,lanebus.RFM_LINEF_RB,lanebus.RFM_LINE_ENTRY_CL,lanebus.RFM_LINE_EXIT_CL,roadbus.RFM_TSR
  Bus Selector30 : BusSelector  OutputSignals=lonbus
  Bus Selector31 : BusSelector  OutputSignals=RFM_BRANCH_LANE,RFM_LEFT_LANE,RFM_CURRENT_LANE,RFM_RIGHT_LANE,RFM_INTERSEC_ALERT,RFM_BRANCH,RFM_REC_LANES
  Bus Selector4 : BusSelector  OutputSignals=VSM_HMI,MRCReq
  Bus Selector5 : BusSelector  OutputSignals=roadbus.RFM_ROAD,roadbus.RFM_UpdateCnt
  Bus Selector6 : BusSelector  OutputSignals=signal1.TOS_LC,signal1.TOS_ACCP0,signal1.TOS_ACCP1,signal1.TOS_ACCP2,signal1.TOS_ACCP3,signal1.TOS_UpdateCnt
  Bus Selector7 : BusSelector  OutputSignals=vxvRefMs,axvRefMs2,axvRoadSlopeMs2,kapTraj
  Bus Selector8 : BusSelector  OutputSignals=EQ4_LAP,EQ4_LH,EQ4_LA,EQ4_LRE
  Bus Selector9 : BusSelector  Commented=on  OutputSignals=DFIM_VSM_STS
  CSA_Pack : Subsystem
  DCT_Pack : Subsystem
  Data Type Conversion : DataTypeConversion  OutDataTypeStr=uint8
  ECM_Pack : Subsystem
  ESP_Pack : Subsystem
  HAP_Pack : Subsystem
  HUT_Pack : Subsystem
  IfALLBus1 : InportShadow  Port=3
  IfVIEBus1 : InportShadow  Port=8
  PLAN : ModelReference  ModelNameDialog=PubIfDecisionPLAN_MDL.slx  SimulationMode=Normal  ModelReferenceVersion=1.158
  Selector : Selector  InputPortWidth=4  IndexOptions=Index vector (dialog)  Indices=1  OutputSizes=1
  Selector1 : Selector  InputPortWidth=4  IndexOptions=Index vector (dialog)  Indices=2  OutputSizes=1
  Selector2 : Selector  InputPortWidth=4  IndexOptions=Index vector (dialog)  Indices=3  OutputSizes=1
  Selector3 : Selector  InputPortWidth=4  IndexOptions=Index vector (dialog)  Indices=4  OutputSizes=1
  Selector4 : Selector  InputPortWidth=2  IndexOptions=Index vector (dialog)  Indices=1  OutputSizes=1
  Selector5 : Selector  InputPortWidth=2  IndexOptions=Index vector (dialog)  Indices=2  OutputSizes=1
  Selector6 : Selector  InputPortWidth=2  IndexOptions=Index vector (dialog)  Indices=1  OutputSizes=1
  Selector7 : Selector  InputPortWidth=2  IndexOptions=Index vector (dialog)  Indices=2  OutputSizes=1
  Subsystem : Subsystem
  Subsystem1 : Subsystem
  Subsystem2 : Subsystem
  Subsystem3 : Subsystem
  Subsystem4 : Subsystem
  Subsystem5 : Subsystem
  Unit Delay{1..4} (4 alike) : UnitDelay  SampleTime=-1  HasFrameUpgradeWarning=on
  VSM : Subsystem
  IfVSMBus : Outport
  IfLSMBus : Outport  Port=2
  IfPlanbus : Outport  Port=3
  wires:
  Bus Creator/1 -> Unit Delay4/1, IfVSMBus/1
  FaultTriggers/1 -> Bus Selector9/1
  IfCANBus/1 -> ECM_Pack/1(In1), DCT_Pack/1(In1), Subsystem4/1(In1), Subsystem3/1(In1), CSA_Pack/1(In1), HAP_Pack/1(In1), Subsystem2/1(In1), HUT_Pack/1(In1), Subsystem1/1(In1), ABM_Pack/1(In1), Subsystem/1(In1), BCM_Pack/1(In1), ESP_Pack/1(In1)
  IfDMSBus/1 -> Bus Selector19/1
  IfCALBus/1 -> Bus Selector20/1
  Bus Selector20/1 -> VSM/18(CAL_VSM_CONFIG)  "<CAL_VSM_CONFIG>"
  Bus Selector9/1 -> ?  "<DFIM_VSM_STS>"
  IfVIEBus/1 -> [IfVIEBus], Bus Selector23/1
  Bus Selector24/4 -> Unit Delay1/1  "<LATC_IFCAngCmdReqValue>"
  Bus Selector24/5 -> Data Type Conversion/1  "<LATC_IFCFuncAngCmdReqFlag>"
  Subsystem5/1(LSM_TJA_ICA) -> Bus Creator9/1  "LSM_TJA_ICA"
  Bus Selector1/1 -> Subsystem5/1(TOS_P0_TARGET_LINE)  "<TOS_P0_TARGET_LINE>"
  Subsystem5/2(LSM_LCK) -> Bus Creator9/2  "LSM_LCK"
  Bus Selector4/1 -> Subsystem5/2(VSM_HMI)  "<VSM_HMI>"
  IfEQ4Bus/1 -> Bus Selector8/1
  Subsystem5/3(LSM_HWA) -> Bus Creator9/3  "LSM_HWA"
  IfALLBus1/1 -> Bus Selector3/1, Bus Selector5/1, Bus Selector1/1
  Bus Creator9/1 -> Bus Selector10/1, Bus Selector29/1, Bus Selector/1, IfLSMBus/1  "IfLSMBus"
  Subsystem5/4(LSM_ESS) -> Bus Creator9/4  "LSM_ESS"
  Subsystem5/5(LSM_UpdateCnt) -> Bus Creator9/5  "LSM_UpdateCnt"
  [IfVSMBus] -> Bus Selector4/1
  IfVIEBus1/1 -> Bus Selector2/1
  ESP_Pack/1(VSM_VCAN_ESP) -> [ESP_Pack], VSM/4(VSM_VCAN_ESP)
  Bus Selector19/1 -> VSM/17(DriverSts)  "<DriverSts>"
  Bus Selector21/1 -> VSM/20(RFM_LINE_L1)  "<RFM_LINE_L1>"
  Bus Selector21/2 -> VSM/21(RFM_LINE_R1)  "<RFM_LINE_R1>"
  Bus Selector21/3 -> VSM/22(RFM_LINE_LB)  "<RFM_LINE_LB>"
  Bus Selector21/4 -> VSM/23(RFM_LINE_RB)  "<RFM_LINE_RB>"
  Bus Selector/1 -> VSM/24(LSM_UpdateCnt)  "<LSM_UpdateCnt>"
  Bus Selector/2 -> VSM/25(LSM_TJA_ICA)  "<LSM_TJA_ICA>"
  Bus Selector/3 -> VSM/26(LSM_HWA)  "<LSM_HWA>"
  Bus Selector/4 -> VSM/27(LSM_LCK)  "<LSM_LCK>"
  Bus Selector/5 -> VSM/28(LSM_ESS)  "<LSM_ESS>"
  Bus Selector25/1 -> VSM/29(TOS_ACCP0)  "<TOS_ACCP0>"
  Bus Selector25/2 -> VSM/30(TOS_AEB_LONOBJ)  "<TOS_AEB_LONOBJ>"
  Bus Selector25/3 -> VSM/31(TOS_ELK)  "<TOS_ELK>"
  Bus Selector25/4 -> VSM/32(TOS_LCKIE)  "<TOS_LCKIE>"
  Bus Selector22/1 -> ?  "<EHRV2_HDR>"
  Bus Selector22/2 -> ?  "<EHRV2_ROAD_ROI>"
  Bus Selector22/3 -> ?  "<EHRV2_ROAD_INFO>"
  Bus Selector23/1 -> VSM/38(axvRefMs2)  "<axvRefMs2>"
  Bus Selector23/2 -> VSM/39(vxvRefMs)  "<vxvRefMs>"
  Bus Selector23/3 -> VSM/40(axvRoadSlopeMs2)  "<axvRoadSlopeMs2>"
  Bus Selector23/4 -> VSM/41(psiDtOpt)  "<axRefDt>"
  Bus Selector23/5 -> VSM/42(ayvRefMs2)  "<ayvRefMs2>"
  Bus Selector23/6 -> VSM/43(kapTraj)  "<kapTraj>"
  Bus Selector24/1 -> VSM/44(AEB_IPHUT_INFO)  "<AEB_IPHUT_INFO>"
  Bus Selector24/2 -> VSM/45(AEB_BRK_INFO)  "<AEB_BRK_INFO>"
  Bus Selector24/3 -> VSM/46(RFM_TSR)  "<RFM_TSR>"
  Unit Delay1/1 -> VSM/47(LATC_IFCTrqOvlCmdReqValue)
  Unit Delay2/1 -> VSM/48(LATC_IFCFuncTrqCmdReqFlag)
  VSM/1(VSM_LON_CTRL) -> Bus Creator/1  "VSM_LON_CTRL"
  VSM/2(VSM_LAT_CTRL) -> Bus Creator/2  "VSM_LAT_CTRL"
  VSM/3(VSM_HMI) -> Bus Creator/3  "VSM_HMI"
  VSM/4(VSM_CTRL_LINE) -> Bus Creator/4  "VSM_CTRL_LINE"
  VSM/5(VSM_TSR) -> Bus Creator/5  "VSM_TSR"
  VSM/6(VSM_TSR_REMAIN) -> Bus Creator/6  "VSM_TSR_REMAIN"
  VSM/8(DataCLCT) -> Bus Creator/8  "DangerPlausMatrix"
  HAP_Pack/1(VSM_VCAN_HAP) -> VSM/16(VSM_VCAN_HAP)
  HUT_Pack/1(VSM_VCAN_HUT) -> VSM/13(VSM_VCAN_HUT)
  ABM_Pack/1(VSM_VCAN_ABM) -> VSM/11(VSM_VCAN_ABM)
  CSA_Pack/1(VSM_VCAN_CSA) -> VSM/10(VSM_VCAN_CSA)
  ECM_Pack/1(VSM_VCAN_ECM) -> VSM/1(VSM_VCAN_ECM)
  DCT_Pack/1(VSM_VCAN_DCT) -> VSM/2(VSM_VCAN_DCT)
  BCM_Pack/1(VSM_VCAN_BCM) -> VSM/7(VSM_VCAN_BCM)
  Subsystem3/1(VSM_VCAN_PBOX) -> VSM/9(VSM_VCAN_PBOX)
  [IfVIEBus] -> Bus Selector7/1
  [IfVSMBus] -> Bus Selector12/1
  IfEHRBus/1 -> Bus Selector22/1
  PLAN/1 -> Bus Creator1/1  "PLAN_DPC_ESS"
  PLAN/2 -> Bus Creator1/2  "PLAN_ALC_DECS"
  PLAN/3 -> Bus Creator1/3
  Bus Creator1/1 -> IfPlanbus/1, [IfPlanbus]
  [IfPlanbus] -> Unit Delay3/1
  Unit Delay3/1 -> Bus Selector14/1
  Bus Selector14/1 -> Subsystem5/6(PLAN_ALC_DECS)  "<PLAN_ALC_DECS>"
  Unit Delay4/1 -> [IfVSMBus]
  [IfPlanbus] -> Bus Selector16/1
  [IfVSMBus] -> Bus Selector18/1
  Bus Selector27/1 -> PLAN/1  "<RFM_LINE_L1>"
  Bus Selector27/2 -> PLAN/2  "<RFM_LINE_R1>"
  Bus Selector10/1 -> PLAN/4  "<LSM_HWA>"
  Bus Selector10/2 -> PLAN/5  "<LSM_ESS>"
  Bus Selector10/3 -> PLAN/6  "<LSM_UpdateCnt>"
  Bus Selector6/1 -> PLAN/7  "<TOS_LC>"
  Bus Selector6/2 -> PLAN/8  "<TOS_ACCP0>"
  Bus Selector6/3 -> PLAN/9  "<TOS_ACCP1>"
  Bus Selector6/4 -> PLAN/10  "<TOS_ACCP2>"
  Bus Selector6/5 -> PLAN/11  "<TOS_ACCP3>"
  Bus Selector6/6 -> PLAN/12  "<TOS_UpdateCnt>"
  Bus Selector27/3 -> PLAN/3  "<RFM_TSR>"
  Bus Selector12/1 -> PLAN/13  "<VSM_LON_CTRL>"
  Bus Selector30/1 -> Bus Selector28/1  "<lonbus>"
  Bus Selector7/1 -> PLAN/14  "<vxvRefMs>"
  Bus Selector7/2 -> PLAN/15  "<axvRefMs2>"
  Bus Selector7/3 -> PLAN/16  "<axvRoadSlopeMs2>"
  Bus Selector7/4 -> PLAN/17  "<kapTraj>"
  Subsystem5/6(LSM_PilotTurnSwSts) -> Bus Creator9/6  "LSM_PilotTurnSwSts"
  IfALLBus/1 -> Bus Selector30/1, Bus Selector21/1, Bus Selector24/1, Bus Selector25/1, Bus Selector6/1, Bus Selector27/1
  Subsystem5/7(LSM_PilotSts) -> Bus Creator9/7, VSM/52(LSM_PilotSts)  "LSM_PilotSts"
  VSM/7(VSM_UOM_LC) -> Bus Creator/7  "VSM_UOM_LC_BUS"
  Bus Selector18/1 -> PLAN/19  "<VSM_HMI>"
  Bus Selector18/2 -> PLAN/23  "<VSM_UOM_LC_BUS>"
  RFM_LANES/1 -> Bus Selector31/1
  Bus Selector8/3 -> Bus Selector15/1  "<EQ4_LA>"
  Bus Selector8/4 -> Bus Selector26/1  "<EQ4_LRE>"
  Bus Selector2/1 -> Subsystem5/4(vxvRefMs)  "<vxvRefMs>"
  Bus Selector2/2 -> Subsystem5/5(kapTraj)  "<kapTraj>"
  Bus Selector5/2 -> Subsystem5/8(RFM_UpdateCnt)  "<RFM_UpdateCnt>"
  Bus Selector5/1 -> Subsystem5/7(RFM_ROAD)  "<RFM_ROAD>"
  Bus Selector31/2 -> Subsystem5/10(RFM_LEFT_LANE)  "<RFM_LEFT_LANE>"
  Bus Selector31/3 -> Subsystem5/11(RFM_CURRENT_LANE)  "<RFM_CURRENT_LANE>"
  Bus Selector31/1 -> Subsystem5/9(RFM_BRANCH_LANE)  "<RFM_BRANCH_LANE>"
  Bus Selector31/4 -> Subsystem5/12(RFM_RIGHT_LANE)  "<RFM_RIGHT_LANE>"
  Bus Selector31/5 -> Subsystem5/13(RFM_INTERSEC_ALERT)  "<RFM_INTERSEC_ALERT>"
  Bus Selector31/6 -> Subsystem5/14(RFM_BRANCH)  "<RFM_BRANCH>"
  Bus Selector31/7 -> Subsystem5/15(RFM_REC_LANES)  "<RFM_REC_LANES>"
  Bus Selector3/1 -> Subsystem5/16(RFM_LINE_L1)  "<RFM_LINE_L1>"
  Bus Selector3/2 -> Subsystem5/17(RFM_LINE_R1)  "<RFM_LINE_R1>"
  Bus Selector3/3 -> Subsystem5/18(RFM_LINE_L2)  "<RFM_LINE_L2>"
  Bus Selector3/4 -> Subsystem5/19(RFM_LINE_R2)  "<RFM_LINE_R2>"
  Bus Selector3/5 -> Subsystem5/20(RFM_LINE_L3)  "<RFM_LINE_L3>"
  Bus Selector3/6 -> Subsystem5/21(RFM_LINE_R3)  "<RFM_LINE_R3>"
  Bus Selector3/7 -> Subsystem5/22(RFM_LINE_CL)  "<RFM_LINE_CL>"
  Bus Selector3/8 -> Subsystem5/23(RFM_LINE_LB)  "<RFM_LINE_LB>"
  Bus Selector3/9 -> Subsystem5/24(RFM_LINE_RB)  "<RFM_LINE_RB>"
  Bus Selector3/10 -> Subsystem5/25(RFM_LINE_PRED)  "<RFM_LINE_PRED>"
  Bus Selector3/11 -> Subsystem5/26(RFM_LINEF_LB)  "<RFM_LINEF_LB>"
  Bus Selector3/12 -> Subsystem5/27(RFM_LINEF_RB)  "<RFM_LINEF_RB>"
  Bus Selector3/13 -> Subsystem5/28(RFM_LINE_ENTRY_CL)  "<RFM_LINE_ENTRY_CL>"
  Bus Selector3/14 -> Subsystem5/29(RFM_LINE_EXIT_CL)  "<RFM_LINE_EXIT_CL>"
  Bus Selector29/1 -> PLAN/21  "<LSM_PilotSts>"
  Bus Selector29/2 -> PLAN/22  "<LSM_PilotTurnSwSts>"
  Bus Selector28/1 -> PLAN/20  "<LONC_VLC_InternalAcc>"
  [ESP_Pack] -> PLAN/18
  PLAN/4 -> Bus Creator1/4  "PLAN_HMI"
  PLAN/5 -> Bus Creator1/5
  PLAN/6 -> Bus Creator1/6
  Bus Selector16/4 -> VSM/54(PLAN_DPC_ESS)  "<PLAN_DPC_ESS>"
  Bus Selector16/3 -> VSM/53(PLAN_ALC_Decision)  "<PLAN_ALC_DECS>"
  Bus Selector16/2 -> VSM/51(PLAN_DriverOffConditionFulfilled)  "<PLAN_DriverOffConditionFulfilled>"
  Bus Selector16/1 -> VSM/50(PLAN_ACCPLAN)  "<PLAN_ACCPLAN>"
  Subsystem5/8(LSM_PilotNohExitDist) -> Bus Creator3/1
  Subsystem5/9(LSM_PilotSPLDist) -> Bus Creator3/2
  Subsystem5/10(LSM_PilotSPL) -> Bus Creator3/3
  Subsystem5/11(LSM_PilotRoadSts) -> Bus Creator3/4  "LSM_PilotRoadSts"
  Bus Creator3/1 -> Bus Selector13/1
  Bus Selector13/1 -> PLAN/24  "<LSM_PilotSPLDist>"
  Bus Selector13/2 -> PLAN/25  "<LSM_PilotSPL>"
  PLAN/7 -> Bus Creator1/7  "PLAN_NOH_SetSpdAdjReq"
  PLAN/8 -> Bus Creator1/8  "PLAN_NOH_SetSpdAdjVal"
  Bus Selector16/5 -> VSM/55(PLAN_NOH_SetSpdAdjReq)  "<PLAN_NOH_SetSpdAdjReq>"
  Bus Selector16/6 -> VSM/56(PLAN_NOH_SetSpdAdjVal)  "<PLAN_NOH_SetSpdAdjVal>"
  Bus Selector13/3 -> PLAN/26  "<LSM_PilotRoadSts>"
  ESP_Pack/2(VSM_VCAN_EPS) -> VSM/5(VSM_VCAN_EPS)
  ESP_Pack/3(VSM_VCAN_PEPS) -> VSM/6(VSM_VCAN_PEPS)
  Subsystem/1(<ACAmbTemp>) -> VSM/8(VSM_ACAmbTemp)
  Subsystem1/1(<IP_VehSpdUnit>) -> VSM/12(VSM_VCAN_IP)
  HUT_Pack/2(VSM_VCAN_CR) -> VSM/14(VSM_VCAN_CR)
  Subsystem2/1(<HighBeamSts_HC>) -> VSM/15(VSM_VCAN_HC)
  Subsystem4/1(Out1) -> VSM/3(VSM_VCAN_HCU)
  Bus Selector15/1 -> Selector/1, Selector1/1, Selector3/1, Selector2/1  "<EQ4_LA_ELEM>"
  Bus Selector15/2 -> Subsystem5/33(EQ4_LA_HDR)  "<EQ4_LA_HDR>"
  Bus Selector8/2 -> Bus Selector17/1  "<EQ4_LH>"
  Bus Selector17/1 -> Selector5/1, Selector4/1  "<EQ4_LH_ELEM>"
  Bus Selector17/2 -> Subsystem5/30(EQ4_LH_HDR)  "<EQ4_LH_HDR>"
  Selector4/1 -> Subsystem5/31(EQ4_LH_ELEM)
  Selector5/1 -> Subsystem5/32(EQ4_LH_ELEM1)
  Selector/1 -> Subsystem5/34(EQ4_LA_ELEM)
  Selector1/1 -> Subsystem5/35(EQ4_LA_ELEM1)
  Selector2/1 -> Subsystem5/36(EQ4_LA_ELEM2)
  Selector3/1 -> Subsystem5/37(EQ4_LA_ELEM3)
  Bus Selector26/2 -> Subsystem5/38(EQ4_LRE_HDR)  "<EQ4_LRE_HDR>"
  Bus Selector26/1 -> Selector7/1, Selector6/1  "<EQ4_LRE_ELEM>"
  Selector6/1 -> Subsystem5/39(EQ4_LRE_ELEM)
  Selector7/1 -> Subsystem5/40(EQ4_LRE_ELEM1)
  Bus Selector3/15 -> Subsystem5/41(RFM_TSR)  "<RFM_TSR>"
  Data Type Conversion/1 -> Unit Delay2/1
  VSM/9(VSM_MRCReq) -> Bus Creator/9
  Bus Selector18/3 -> PLAN/29  "<MRCReq>"
  Bus Selector4/2 -> Subsystem5/3(VSM_ReqMRC)  "<MRCReq>"
  Subsystem5/12(LSM_TJALineSource) -> VSM/57(LSM_TJALineSource)

== system Noa_Nofusion_angle/SensorDia ==
  function : TriggerPort  TriggerType=function-call  VariantControl=Variant
  AND : Logic  Inputs=8  IconShape=distinctive  AllPortsSameDT=off  OutDataTypeStr=boolean
  Bus Selector : BusSelector  OutputSignals=RSDS_L_hdr_TimerStempStatus Value,RSDS_R_hdr_TimerStempStatus Value,CR_L_hdr_TimerStempStatus Value,CR_R_hdr_TimerStempStatus Value,RSDS_L_hdr_ErrorStatus Value,RSDS_R_hdr_ErrorStatus Value,CR_L_hdr_ErrorStatus Value,CR_R_hdr_ErrorStatus Value
  CR_Dia : dsmpblib/Data Inport  Priority=10000
      settings: SourceProductName=dSPACE Model Interface Blockset
  Compare To Constant{,1..3} (4 alike) : simulink/Logic and Bit Operations/Compare To Constant  relop===  const=8  OutDataTypeStr=boolean
  Compare To Constant{4..7} (4 alike) : simulink/Logic and Bit Operations/Compare To Constant  relop===  const=0  OutDataTypeStr=boolean
  Signal Copy{,1..7} (8 alike) : SignalConversion  OverrideOpt=off
  Source_Dia_CRsts : Outport
  wires:
  Signal Copy6/1 -> Compare To Constant6/1  "Source_Dia_ErrorStatusCRL"
  Compare To Constant2/1 -> AND/3
  Compare To Constant7/1 -> AND/8
  Bus Selector/7 -> Signal Copy6/1  "<CR_L_hdr_ErrorStatus Value>"
  Compare To Constant6/1 -> AND/7
  AND/1 -> Source_Dia_CRsts/1  "Source_Dia_CRsts"
  Compare To Constant4/1 -> AND/5
  Compare To Constant/1 -> AND/1
  Compare To Constant5/1 -> AND/6
  Signal Copy4/1 -> Compare To Constant4/1  "Source_Dia_ErrorStatusRSDSL"
  Bus Selector/1 -> Signal Copy/1  "<RSDS_L_hdr_TimerStempStatus Value>"
  Signal Copy/1 -> Compare To Constant/1  "Source_Dia_TimeSnycStsRSDSL"
  Signal Copy3/1 -> Compare To Constant3/1  "Source_Dia_TimeSnycStsCRR"
  Compare To Constant1/1 -> AND/2
  Signal Copy1/1 -> Compare To Constant1/1  "Source_Dia_TimeSnycStsRSDSR"
  Compare To Constant3/1 -> AND/4
  Signal Copy5/1 -> Compare To Constant5/1  "Source_Dia_ErrorStatusRSDSR"
  Bus Selector/6 -> Signal Copy5/1  "<RSDS_R_hdr_ErrorStatus Value>"
  Signal Copy2/1 -> Compare To Constant2/1  "Source_Dia_TimeSnycStsCRL"
  Bus Selector/5 -> Signal Copy4/1  "<RSDS_L_hdr_ErrorStatus Value>"
  Bus Selector/8 -> Signal Copy7/1  "<CR_R_hdr_ErrorStatus Value>"
  Bus Selector/3 -> Signal Copy2/1  "<CR_L_hdr_TimerStempStatus Value>"
  Bus Selector/4 -> Signal Copy3/1  "<CR_R_hdr_TimerStempStatus Value>"
  Bus Selector/2 -> Signal Copy1/1  "<RSDS_R_hdr_TimerStempStatus Value>"
  CR_Dia/1 -> Bus Selector/1
  Signal Copy7/1 -> Compare To Constant7/1  "Source_Dia_ErrorStatusCRR"

== system Noa_Nofusion_angle/SimBCM ==
  VCAN : Inport
  PLAN_ALC_DECS : Inport  Port=2
  function : TriggerPort  TriggerType=function-call  VariantControl=Variant
  BCMsim : MATLAB Function  TreatAsAtomicUnit=on
  Bus Selector : BusSelector  OutputSignals=PLAN_ALC_DECS.PLAN_ALC_TurnLightReq
  Bus Selector3 : BusSelector  OutputSignals=CSA_NODE.CSA2_MSG.SteerWheelAngSign,CSA_NODE.CSA2_MSG.SteerWheelAng,CSA_NODE.CSA1_MSG.LTurnLmpSwtSts,CSA_NODE.CSA1_MSG.RTurnLmpSwtSts
  CSALampCtrlSim : Subsystem
  LTurnLmpSwtSts : Outport
  RTurnLmpSwtSts : Outport  Port=2
  CSASim_IDC_L2_LampReq : Outport  Port=3
  wires:
  CSALampCtrlSim/1(LTurnLmpSwtSts) -> LTurnLmpSwtSts/1, BCMsim/1(SimLeLmp)
  CSALampCtrlSim/2(RTurnLmpSwtSts) -> RTurnLmpSwtSts/1, BCMsim/2(SimRiLmp)
  Bus Selector/1 -> CSALampCtrlSim/5(IDC_L2_LampReq), BCMsim/3(Model_IDC_L2_LampReq)  "<PLAN_ALC_TurnLightReq>"
  BCMsim/1(CSASim_LampReq) -> CSASim_IDC_L2_LampReq/1
  PLAN_ALC_DECS/1 -> Bus Selector/1
  Bus Selector3/3 -> CSALampCtrlSim/3(LeLmp)  "<LTurnLmpSwtSts>"
  Bus Selector3/2 -> CSALampCtrlSim/2(SteerWheelAngSign)  "<SteerWheelAng>"
  Bus Selector3/4 -> CSALampCtrlSim/4(RiLmp)  "<RTurnLmpSwtSts>"
  Bus Selector3/1 -> CSALampCtrlSim/1(SteerWheelAng)  "<SteerWheelAngSign>"
  VCAN/1 -> Bus Selector3/1

== system Noa_Nofusion_angle/Subsystem1 ==
  note: crtype
  l3_RFMResult : Inport
  road : Inport  Port=2
  lane : Inport  Port=3
  LSMback : Inport  Port=4
  Bus Assignment5 : BusAssignment  AssignedSignals=RFM_ROAD.nLaneNum,RFM_ROAD.b_toll,RFM_ROAD.i_mapvalid,RFM_TSR.RoadType
  Bus Assignment6 : BusAssignment  AssignedSignals=RFM_INTERSEC_ALERT.b_is_available,RFM_INTERSEC_ALERT.f_distance,RFM_INTERSEC_ALERT.en_direction,RFM_INTERSEC_ALERT.en_type,RFM_BRANCH.f_turning_angle,RFM_BRANCH.en_RoadClass,RFM_RIGHT_LANE.en_lane_type,RFM_RIGHT_LANE.b_is_avalible,RFM_CURRENT_LANE.en_lane_type,RFM_CURRENT_LANE.b_is_avalible
  Bus Selector : BusSelector  OutputSignals=b_is_available,f_distance,en_direction,en_type,st_branch.f_turning_angle
  Bus Selector1 : BusSelector  OutputSignals=i_lane_number
  Bus Selector2 : BusSelector  OutputSignals=st_intersec_alert,st_road_info,st_lanes
  Bus Selector3 : BusSelector  OutputSignals=en_road_type,ast_lane_number_vec,b_toll
  Bus Selector4 : BusSelector  OutputSignals=LSM_HWA.MRiLane
  Bus Selector5 : BusSelector  OutputSignals=en_lane_type
  Bus Selector8 : BusSelector  OutputSignals=en_lane_type
  Constant : Constant  Value=P_RFM_mapvalid
  Constant1 : Constant  Value=5  OutDataTypeStr=uint8
  Constant2 : Constant  Value=0  OutDataTypeStr=uint8
  Constant3 : Constant  OutDataTypeStr=uint8
  Constant4 : Constant  Value=P_RFM_RoadType  OutDataTypeStr=uint8
  Constant6 : Constant  Value=0  OutDataTypeStr=uint8
  Selector1 : Selector  InputPortWidth=3  IndexOptions=Index vector (dialog)  Indices=1  OutputSizes=1
  Selector5 : Selector  InputPortWidth=3  IndexOptions=Index vector (dialog)  Indices=2  OutputSizes=1
  Selector6 : Selector  InputPortWidth=3  IndexOptions=Index vector (dialog)  Indices=3  OutputSizes=1
  Switch : Switch  Criteria=u2 ~= 0
  Switch1 : Switch  Criteria=u2 ~= 0
  Terminator : Terminator
  Terminator1 : Terminator
  IfRFM_LANES_In : Outport
  roadbus : Outport  Port=2
  wires:
  Bus Selector2/1 -> Bus Selector/1  "<st_intersec_alert>"
  Bus Selector/5 -> Bus Assignment6/6  "<f_turning_angle>"
  Bus Selector3/3 -> Bus Assignment5/3  "<b_toll>"
  Selector5/1 -> Bus Selector5/1
  Bus Selector1/1 -> Bus Assignment5/2  "<i_lane_number>"
  Bus Selector/1 -> Bus Assignment6/2  "<b_is_available>"
  Bus Selector2/3 -> Selector6/1, Selector5/1  "<st_lanes>"
  Bus Selector3/1 -> Bus Assignment6/7  "<en_road_type>"
  Bus Selector2/2 -> Bus Selector3/1  "<st_road_info>"
  Selector6/1 -> Bus Selector8/1
  Bus Assignment5/1 -> roadbus/1
  Bus Selector/4 -> Bus Assignment6/5  "<en_type>"
  Bus Assignment6/1 -> IfRFM_LANES_In/1
  Bus Selector/2 -> Bus Assignment6/3  "<f_distance>"
  Bus Selector/3 -> Bus Assignment6/4  "<en_direction>"
  l3_RFMResult/1 -> Bus Selector2/1
  road/1 -> Bus Assignment5/1
  lane/1 -> Bus Assignment6/1
  Bus Selector5/1 -> Terminator1/1  "<en_lane_type>"
  Bus Selector8/1 -> Terminator/1  "<en_lane_type>"
  Bus Selector3/2 -> Selector1/1  "<ast_lane_number_vec>"
  Selector1/1 -> Bus Selector1/1
  Constant/1 -> Bus Assignment5/4
  Constant4/1 -> Bus Assignment5/5
  LSMback/1 -> Bus Selector4/1
  Bus Selector4/1 -> Switch/2, Switch1/2  "<MRiLane>"
  Switch/1 -> Bus Assignment6/10
  Constant1/1 -> Switch/1
  Constant2/1 -> Switch/3
  Constant3/1 -> Bus Assignment6/11, Switch1/3
  Switch1/1 -> Bus Assignment6/9
  Constant6/1 -> Switch1/1, Bus Assignment6/8

== system Noa_Nofusion_angle/Subsystem3 ==
  function : TriggerPort  TriggerType=function-call  VariantControl=Variant
  Compare To Constant : simulink/Logic and Bit Operations/Compare To Constant  relop===  const=1344  OutDataTypeStr=boolean
  S-Function1 : S-Function  FunctionName=sfun_roadfus_L3  SFunctionDeploymentMode=off  EnableBusSupport=off
  Subsystem2 : Subsystem
  UDP Receive (3) : dsmpblib/Data Inport  Priority=10000
      settings: SourceProductName=dSPACE Model Interface Blockset
  Out2 : Outport
  wires:
  Compare To Constant/1 -> Subsystem2/Enable
  Subsystem2/1(Out1) -> S-Function1/1
  UDP Receive (3)/3 -> Compare To Constant/1
  UDP Receive (3)/1 -> Subsystem2/1(In1)
  S-Function1/1 -> Out2/1
